simulink model "CF012A_GmStrtStop"  (R2013b)
settings: Solver=FixedStepDiscrete  SolverMode=SingleTasking  StartTime=0.0  StopTime=1  FixedStep=0.002  RelTol=1e-3
values from neighbouring files (symbols this model uses):
  CNV100MICROSECTOMILLISEC_MILLISECPERCNT_F32 = DataDict.Constant    [CF012A_GmStrtStop_DataDict.m]
  DISMOD_CNT_U08 = DataDict.Constant    [CF012A_GmStrtStop_DataDict.m]
  DISMODRATE_ULSPERSEC_F32 = DataDict.Constant    [CF012A_GmStrtStop_DataDict.m]
  FLTMOD_CNT_U08 = DataDict.Constant    [CF012A_GmStrtStop_DataDict.m]
  GmStrtStopEna = DataDict.Calibration    [CF012A_GmStrtStop_DataDict.m]
  GmStrtStopFltRateLim = DataDict.Calibration    [CF012A_GmStrtStop_DataDict.m]
  GmStrtStopMod1ToStopRateLim = DataDict.Calibration    [CF012A_GmStrtStop_DataDict.m]
  GmStrtStopNormRateLim = DataDict.Calibration    [CF012A_GmStrtStop_DataDict.m]
  GmStrtStopNormToMod1RateLim = DataDict.Calibration    [CF012A_GmStrtStop_DataDict.m]
  GmStrtStopStopAndMod2RateLim = DataDict.Calibration    [CF012A_GmStrtStop_DataDict.m]
  GmStrtStopStopMod1Tmr = DataDict.Calibration    [CF012A_GmStrtStop_DataDict.m]
  GmStrtStopStopMod2Tmr = DataDict.Calibration    [CF012A_GmStrtStop_DataDict.m]
  MOD1_CNT_U08 = DataDict.Constant    [CF012A_GmStrtStop_DataDict.m]
  MOD2_CNT_U08 = DataDict.Constant    [CF012A_GmStrtStop_DataDict.m]
  NORMMOD_CNT_U08 = DataDict.Constant    [CF012A_GmStrtStop_DataDict.m]
  STOPMOD_CNT_U08 = DataDict.Constant    [CF012A_GmStrtStop_DataDict.m]
  STRTSTOPRATEHILIM_ULSPERSEC_F32 = DataDict.Constant    [CF012A_GmStrtStop_DataDict.m]
  STRTSTOPRATELOWRLIM_ULSPERSEC_F32 = DataDict.Constant    [CF012A_GmStrtStop_DataDict.m]
  STRTSTOPSCAHILIM_ULS_F32 = DataDict.Constant    [CF012A_GmStrtStop_DataDict.m]
  STRTSTOPSCALOWRLIM_ULS_F32 = DataDict.Constant    [CF012A_GmStrtStop_DataDict.m]
undefined symbols (not defined in the file or in its folder): u2, u3, u4, u5
libraries: FixdToFloat x2, NxtrLim x2, simulink x2
(part 4 of 4)

== system CF012A_GmStrtStop/GmStrtStop/GmStrtStopPer1/Inter1ToStopModFlg/RefTi ==
  Action Port : ActionPort  ActionType=else
  Constant13 : Constant  RequirementInfo={} %GIDa_ee595446_fddf_49fb_8bdf_b7998be5b5f2  Value=false  OutDataTypeStr=boolean
      settings: AttributesFormatString=%<OutDataTypeStr>
  CopyRight2 : Subsystem  Description=|  mask(Copyright Information){none=on}
      | Copyright info block.                                               
      |                                                                     
      | Place copyright information at the top of every subsystem in design.
      mask prompts: none "No parameters"
      mask help: Place copyright information at the top of every subsystem in design.
      mask Display:
      | NxtrConf = 'Nexteer Confidential';
      | 
      | sys = bdroot; %handle for the current model ("system")
      | first = get_param(sys,'Created');
      | if(isempty(first))
      |     first = datestr(now,'yyyy');
      | else
      |     first = first(end-3:end);  %year is last four digits
      | end
      | 
      | last = get_param(sys,'LastModifiedDate');
      | if isempty(last)
      |     last = datestr(now,'yyyy');
      | else
      |     last = last(end-3:end);
      | end
      | 
      | if strcmp(first,last)
      |     fprintf('%s -- Copyright %s Nexteer',NxtrConf,first)
      | else
      |     fprintf('%s -- %s%s- %s Nexteer',NxtrConf,char(169),first,last)
      | end
  Data Store Write9 : DataStoreWrite  DataStoreName=Mod1RefTmr
  GetRefTmr100MicroSec32bit : Subsystem
  TmrElpsdThd : Outport
  wires:
  GetRefTmr100MicroSec32bit/1(RefTmr) -> Data Store Write9/1
  Constant13/1 -> TmrElpsdThd/1

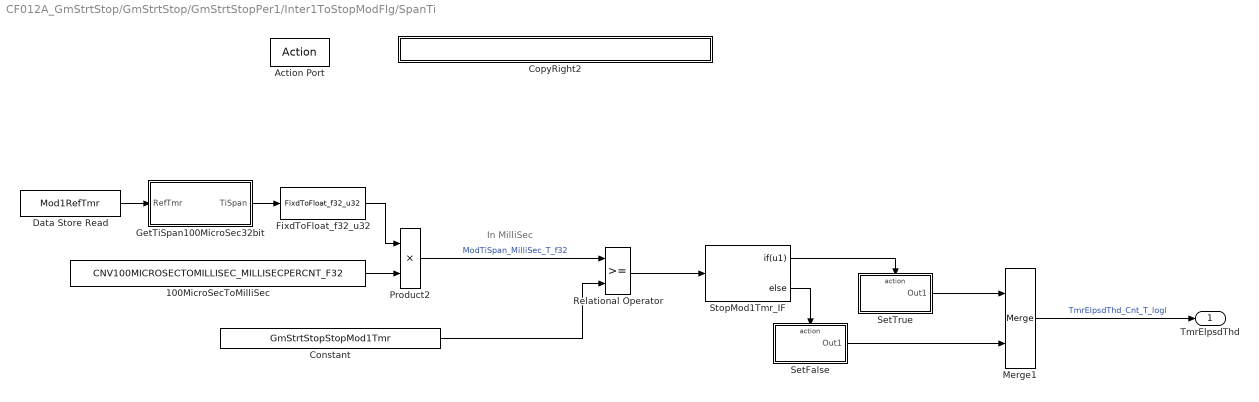
== system CF012A_GmStrtStop/GmStrtStop/GmStrtStopPer1/Inter1ToStopModFlg/SpanTi ==
  note: In MilliSec
  Action Port : ActionPort  ActionType=then
  100MicroSecToMilliSec : Constant  RequirementInfo="{'linktype_rmi_doors' '0000c6e0 (/GM T1XX/SubSystem Specifications/Customer Functions/CF012 12V Start Stop)' '#149' 'true' 'REQ:  149' '' } %GIDa_f27a5255_6b96_489d_8647_639b65e7e1e3"  Value=CNV100MICROSECTOMILLISEC_MILLISECPERCNT_F32
  Constant : Constant  RequirementInfo="{'linktype_rmi_doors' '0000c6e0 (/GM T1XX/SubSystem Specifications/Customer Functions/CF012 12V Start Stop)' '#149' 'true' 'REQ:  149' '' } %GIDa_161a89a7_a936_46ad_9e50_4b6beac1caa8"  Value=GmStrtStopStopMod1Tmr
  CopyRight2 : Subsystem  Description=|  mask(Copyright Information){none=on}
      | Copyright info block.                                               
      |                                                                     
      | Place copyright information at the top of every subsystem in design.
      mask prompts: none "No parameters"
      mask help: Place copyright information at the top of every subsystem in design.
      mask Display:
      | NxtrConf = 'Nexteer Confidential';
      | 
      | sys = bdroot; %handle for the current model ("system")
      | first = get_param(sys,'Created');
      | if(isempty(first))
      |     first = datestr(now,'yyyy');
      | else
      |     first = first(end-3:end);  %year is last four digits
      | end
      | 
      | last = get_param(sys,'LastModifiedDate');
      | if isempty(last)
      |     last = datestr(now,'yyyy');
      | else
      |     last = last(end-3:end);
      | end
      | 
      | if strcmp(first,last)
      |     fprintf('%s -- Copyright %s Nexteer',NxtrConf,first)
      | else
      |     fprintf('%s -- %s%s- %s Nexteer',NxtrConf,char(169),first,last)
      | end
  Data Store Read : DataStoreRead  RequirementInfo="{'linktype_rmi_doors' '0000c6e0 (/GM T1XX/SubSystem Specifications/Customer Functions/CF012 12V Start Stop)' '#149' 'true' 'REQ:  149' '' } %GIDa_f243752d_cd64_4ade_bc30_06d78740bec9"  DataStoreName=Mod1RefTmr
  FixdToFloat_f32_u32 : FixdToFloat/FixdToFloat_f32_u32  RequirementInfo="{'linktype_rmi_doors' '0000c6e0 (/GM T1XX/SubSystem Specifications/Customer Functions/CF012 12V Start Stop)' '#149' 'true' 'REQ:  149' '' } %GIDa_724a14fd_bedc_4ae1_8651_07fb98cb7006"  Param1=0
  GetTiSpan100MicroSec32bit : Subsystem  RequirementInfo="{'linktype_rmi_doors' '0000c6e0 (/GM T1XX/SubSystem Specifications/Customer Functions/CF012 12V Start Stop)' '#149' 'true' 'REQ:  149' '' } %GIDa_42f2edbe_6506_45bf_bc5f_21ff22e5da44"
  Merge1 : Merge  RequirementInfo="{'linktype_rmi_doors' '0000c6e0 (/GM T1XX/SubSystem Specifications/Customer Functions/CF012 12V Start Stop)' '#149' 'true' 'REQ:  149' '' } %GIDa_b6f22ad7_a1b8_4e7a_82f9_c53496e4294b"
  Product2 : Product  RequirementInfo="{'linktype_rmi_doors' '0000c6e0 (/GM T1XX/SubSystem Specifications/Customer Functions/CF012 12V Start Stop)' '#149' 'true' 'REQ:  149' '' } %GIDa_358ce13a_3b2a_451b_80f1_72e22c5f1708"
  Relational Operator : RelationalOperator  RequirementInfo="{'linktype_rmi_doors' '0000c6e0 (/GM T1XX/SubSystem Specifications/Customer Functions/CF012 12V Start Stop)' '#149' 'true' 'REQ:  149' '' } %GIDa_e7de6d6e_7f4c_4fc6_98dc_b2abb4573d8c"  OutDataTypeStr=boolean
  SetFalse : Subsystem  RequirementInfo="{'linktype_rmi_doors' '0000c6e0 (/GM T1XX/SubSystem Specifications/Customer Functions/CF012 12V Start Stop)' '#149' 'true' 'REQ:  149' '' } %GIDa_d7f0596c_8f68_4a27_b553_110820238b8a"  TreatAsAtomicUnit=on
  SetTrue : Subsystem  RequirementInfo="{'linktype_rmi_doors' '0000c6e0 (/GM T1XX/SubSystem Specifications/Customer Functions/CF012 12V Start Stop)' '#149' 'true' 'REQ:  149' '' } %GIDa_3df73667_32db_41d3_8694_836724889a59"  TreatAsAtomicUnit=on
  StopMod1Tmr_IF : If  RequirementInfo="{'linktype_rmi_doors' '0000c6e0 (/GM T1XX/SubSystem Specifications/Customer Functions/CF012 12V Start Stop)' '#149' 'true' 'REQ:  149' '' } %GIDa_ab1d4f5e_890c_4780_96ee_c57598ab3683"  IfExpression=u1
  TmrElpsdThd : Outport  RequirementInfo="{'linktype_rmi_doors' '0000c6e0 (/GM T1XX/SubSystem Specifications/Customer Functions/CF012 12V Start Stop)' '#149' 'true' 'REQ:  149' '' } %GIDa_6efc0186_5b61_45a8_8aa0_b92fa27113a3"
  wires:
  Data Store Read/1 -> GetTiSpan100MicroSec32bit/1(RefTmr)
  Merge1/1 -> TmrElpsdThd/1  "TmrElpsdThd_Cnt_T_logl"
  GetTiSpan100MicroSec32bit/1(TiSpan) -> FixdToFloat_f32_u32/1
  Relational Operator/1 -> StopMod1Tmr_IF/1
  SetTrue/1(Out1) -> Merge1/1
  SetFalse/1(Out1) -> Merge1/2
  StopMod1Tmr_IF/1 -> SetTrue/Action
  StopMod1Tmr_IF/2 -> SetFalse/Action
  100MicroSecToMilliSec/1 -> Product2/2
  FixdToFloat_f32_u32/1 -> Product2/1
  Product2/1 -> Relational Operator/1  "ModTiSpan_MilliSec_T_f32"
  Constant/1 -> Relational Operator/2

== system CF012A_GmStrtStop/GmStrtStop/GmStrtStopPer1/Inter2ToStopModFlg/CopyRight2 ==

== system CF012A_GmStrtStop/GmStrtStop/GmStrtStopPer1/Inter2ToStopModFlg/RefTi ==
  Action Port : ActionPort  ActionType=else
  Constant13 : Constant  RequirementInfo={} %GIDa_2f60d0b6_d859_47c7_824c_82648ed235eb  Value=false  OutDataTypeStr=boolean
      settings: AttributesFormatString=%<OutDataTypeStr>
  CopyRight2 : Subsystem  Description=|  mask(Copyright Information){none=on}
      | Copyright info block.                                               
      |                                                                     
      | Place copyright information at the top of every subsystem in design.
      mask prompts: none "No parameters"
      mask help: Place copyright information at the top of every subsystem in design.
      mask Display:
      | NxtrConf = 'Nexteer Confidential';
      | 
      | sys = bdroot; %handle for the current model ("system")
      | first = get_param(sys,'Created');
      | if(isempty(first))
      |     first = datestr(now,'yyyy');
      | else
      |     first = first(end-3:end);  %year is last four digits
      | end
      | 
      | last = get_param(sys,'LastModifiedDate');
      | if isempty(last)
      |     last = datestr(now,'yyyy');
      | else
      |     last = last(end-3:end);
      | end
      | 
      | if strcmp(first,last)
      |     fprintf('%s -- Copyright %s Nexteer',NxtrConf,first)
      | else
      |     fprintf('%s -- %s%s- %s Nexteer',NxtrConf,char(169),first,last)
      | end
  Data Store Write9 : DataStoreWrite  DataStoreName=Mod2RefTmr
  GetRefTmr100MicroSec32bit : Subsystem
  TmrElpsdThd : Outport
  wires:
  Constant13/1 -> TmrElpsdThd/1
  GetRefTmr100MicroSec32bit/1(RefTmr) -> Data Store Write9/1

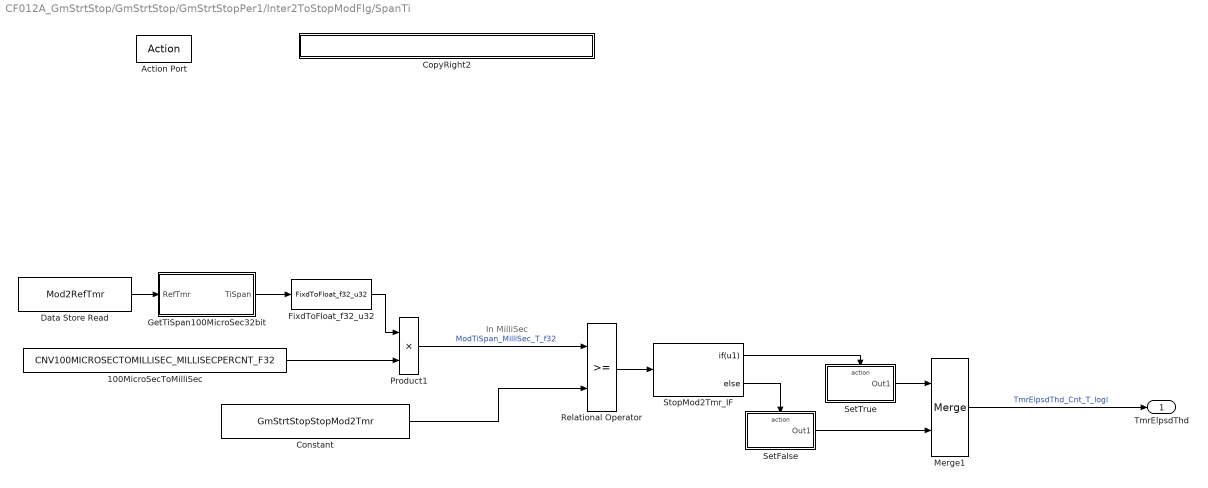
== system CF012A_GmStrtStop/GmStrtStop/GmStrtStopPer1/Inter2ToStopModFlg/SpanTi ==
  note: In MilliSec
  Action Port : ActionPort  ActionType=then
  100MicroSecToMilliSec : Constant  Value=CNV100MICROSECTOMILLISEC_MILLISECPERCNT_F32
  Constant : Constant  RequirementInfo={} %GIDa_5b9b31eb_6e21_4040_a5c7_63bbbbf883bd  Value=GmStrtStopStopMod2Tmr
  CopyRight2 : Subsystem  Description=|  mask(Copyright Information){none=on}
      | Copyright info block.                                               
      |                                                                     
      | Place copyright information at the top of every subsystem in design.
      mask prompts: none "No parameters"
      mask help: Place copyright information at the top of every subsystem in design.
      mask Display:
      | NxtrConf = 'Nexteer Confidential';
      | 
      | sys = bdroot; %handle for the current model ("system")
      | first = get_param(sys,'Created');
      | if(isempty(first))
      |     first = datestr(now,'yyyy');
      | else
      |     first = first(end-3:end);  %year is last four digits
      | end
      | 
      | last = get_param(sys,'LastModifiedDate');
      | if isempty(last)
      |     last = datestr(now,'yyyy');
      | else
      |     last = last(end-3:end);
      | end
      | 
      | if strcmp(first,last)
      |     fprintf('%s -- Copyright %s Nexteer',NxtrConf,first)
      | else
      |     fprintf('%s -- %s%s- %s Nexteer',NxtrConf,char(169),first,last)
      | end
  Data Store Read : DataStoreRead  DataStoreName=Mod2RefTmr
  FixdToFloat_f32_u32 : FixdToFloat/FixdToFloat_f32_u32  Param1=0
  GetTiSpan100MicroSec32bit : Subsystem
  Merge1 : Merge
  Product1 : Product
  Relational Operator : RelationalOperator  OutDataTypeStr=boolean
  SetFalse : Subsystem  TreatAsAtomicUnit=on
  SetTrue : Subsystem  TreatAsAtomicUnit=on
  StopMod2Tmr_IF : If  IfExpression=u1
  TmrElpsdThd : Outport
  wires:
  StopMod2Tmr_IF/2 -> SetFalse/Action
  SetFalse/1(Out1) -> Merge1/2
  SetTrue/1(Out1) -> Merge1/1
  StopMod2Tmr_IF/1 -> SetTrue/Action
  Relational Operator/1 -> StopMod2Tmr_IF/1
  GetTiSpan100MicroSec32bit/1(TiSpan) -> FixdToFloat_f32_u32/1
  Merge1/1 -> TmrElpsdThd/1  "TmrElpsdThd_Cnt_T_logl"
  Data Store Read/1 -> GetTiSpan100MicroSec32bit/1(RefTmr)
  FixdToFloat_f32_u32/1 -> Product1/1
  100MicroSecToMilliSec/1 -> Product1/2
  Product1/1 -> Relational Operator/1  "ModTiSpan_MilliSec_T_f32"
  Constant/1 -> Relational Operator/2

== system CF012A_GmStrtStop/GmStrtStop/GmStrtStopPer1/PassDtrmnRateRes/CopyRight2 ==

== system CF012A_GmStrtStop/GmStrtStop/GmStrtStopPer1/DtrmnPrevActSt/PassLastSt/CopyRight2 ==

== system CF012A_GmStrtStop/GmStrtStop/GmStrtStopPer1/DtrmnPrevActSt/PassPrevLoopRes/CopyRight2 ==

== system CF012A_GmStrtStop/GmStrtStop/GmStrtStopPer1/DtrmnRateLim/DoNothing/CopyRight2 ==

== system CF012A_GmStrtStop/GmStrtStop/GmStrtStopPer1/DtrmnRateLim/FltMod/CopyRight2 ==

== system CF012A_GmStrtStop/GmStrtStop/GmStrtStopPer1/DtrmnRateLim/Inter1Mod/CopyRight2 ==

== system CF012A_GmStrtStop/GmStrtStop/GmStrtStopPer1/DtrmnRateLim/Inter1Mod/THEN1 ==
  note: Change Log:
      | Oct 12, 2012  Created by Kevin Derry as a 1-input, 1-output block
      | Nov 30, 2012  dynamically configurable for 1 to 5 ports.
  note: Do not modify these blocks manually.  They
      | are generated programatically.  Changing the
      | number of blocks available or their names requires
      | corresponding changes to Callback and Initialization
      | routines.
      |
      | Do not change the "Display" tab of mask editor.  The
      | outport names are created programatically in the
      | "Initialize" section.
  In1 : Inport
  Action Port : ActionPort  ActionType=then
  In{2..5} (4 alike) : Ground
  Out{2..5} (4 alike) : Terminator
  Out1 : Outport
  wires:
  In1/1 -> Out1/1
  In2/1 -> Out2/1
  In3/1 -> Out3/1
  In4/1 -> Out4/1
  In5/1 -> Out5/1

== system CF012A_GmStrtStop/GmStrtStop/GmStrtStopPer1/DtrmnRateLim/Inter1Mod/THEN2 ==
  note: Do not modify these blocks manually.  They
      | are generated programatically.  Changing the
      | number of blocks available or their names requires
      | corresponding changes to Callback and Initialization
      | routines.
      |
      | Do not change the "Display" tab of mask editor.  The
      | outport names are created programatically in the
      | "Initialize" section.
  note: Change Log:
      | Oct 12, 2012  Created by Kevin Derry as a 1-input, 1-output block
      | Nov 30, 2012  dynamically configurable for 1 to 5 ports.
  In1 : Inport
  Action Port : ActionPort  ActionType=elseif
  In{2..5} (4 alike) : Ground
  Out{2..5} (4 alike) : Terminator
  Out1 : Outport
  wires:
  In5/1 -> Out5/1
  In4/1 -> Out4/1
  In3/1 -> Out3/1
  In2/1 -> Out2/1
  In1/1 -> Out1/1

== system CF012A_GmStrtStop/GmStrtStop/GmStrtStopPer1/DtrmnRateLim/Inter1Mod/THEN3 ==
  note: Change Log:
      | Oct 12, 2012  Created by Kevin Derry as a 1-input, 1-output block
      | Nov 30, 2012  dynamically configurable for 1 to 5 ports.
  note: Do not modify these blocks manually.  They
      | are generated programatically.  Changing the
      | number of blocks available or their names requires
      | corresponding changes to Callback and Initialization
      | routines.
      |
      | Do not change the "Display" tab of mask editor.  The
      | outport names are created programatically in the
      | "Initialize" section.
  In1 : Inport
  Action Port : ActionPort  ActionType=else
  In{2..5} (4 alike) : Ground
  Out{2..5} (4 alike) : Terminator
  Out1 : Outport
  wires:
  In1/1 -> Out1/1
  In2/1 -> Out2/1
  In3/1 -> Out3/1
  In4/1 -> Out4/1
  In5/1 -> Out5/1

== system CF012A_GmStrtStop/GmStrtStop/GmStrtStopPer1/DtrmnRateLim/Inter2Mod/CopyRight2 ==

== system CF012A_GmStrtStop/GmStrtStop/GmStrtStopPer1/DtrmnRateLim/Inter2Mod/THEN1 ==
  note: Change Log:
      | Oct 12, 2012  Created by Kevin Derry as a 1-input, 1-output block
      | Nov 30, 2012  dynamically configurable for 1 to 5 ports.
  note: Do not modify these blocks manually.  They
      | are generated programatically.  Changing the
      | number of blocks available or their names requires
      | corresponding changes to Callback and Initialization
      | routines.
      |
      | Do not change the "Display" tab of mask editor.  The
      | outport names are created programatically in the
      | "Initialize" section.
  In1 : Inport
  Action Port : ActionPort  ActionType=then
  In{2..5} (4 alike) : Ground
  Out{2..5} (4 alike) : Terminator
  Out1 : Outport
  wires:
  In1/1 -> Out1/1
  In2/1 -> Out2/1
  In3/1 -> Out3/1
  In4/1 -> Out4/1
  In5/1 -> Out5/1

== system CF012A_GmStrtStop/GmStrtStop/GmStrtStopPer1/DtrmnRateLim/Inter2Mod/THEN2 ==
  note: Do not modify these blocks manually.  They
      | are generated programatically.  Changing the
      | number of blocks available or their names requires
      | corresponding changes to Callback and Initialization
      | routines.
      |
      | Do not change the "Display" tab of mask editor.  The
      | outport names are created programatically in the
      | "Initialize" section.
  note: Change Log:
      | Oct 12, 2012  Created by Kevin Derry as a 1-input, 1-output block
      | Nov 30, 2012  dynamically configurable for 1 to 5 ports.
  In1 : Inport
  Action Port : ActionPort  ActionType=elseif
  In{2..5} (4 alike) : Ground
  Out{2..5} (4 alike) : Terminator
  Out1 : Outport
  wires:
  In5/1 -> Out5/1
  In4/1 -> Out4/1
  In3/1 -> Out3/1
  In2/1 -> Out2/1
  In1/1 -> Out1/1

== system CF012A_GmStrtStop/GmStrtStop/GmStrtStopPer1/DtrmnRateLim/Inter2Mod/THEN3 ==
  note: Change Log:
      | Oct 12, 2012  Created by Kevin Derry as a 1-input, 1-output block
      | Nov 30, 2012  dynamically configurable for 1 to 5 ports.
  note: Do not modify these blocks manually.  They
      | are generated programatically.  Changing the
      | number of blocks available or their names requires
      | corresponding changes to Callback and Initialization
      | routines.
      |
      | Do not change the "Display" tab of mask editor.  The
      | outport names are created programatically in the
      | "Initialize" section.
  In1 : Inport
  Action Port : ActionPort  ActionType=else
  In{2..5} (4 alike) : Ground
  Out{2..5} (4 alike) : Terminator
  Out1 : Outport
  wires:
  In1/1 -> Out1/1
  In2/1 -> Out2/1
  In3/1 -> Out3/1
  In4/1 -> Out4/1
  In5/1 -> Out5/1

== system CF012A_GmStrtStop/GmStrtStop/GmStrtStopPer1/DtrmnRateLim/NormMod/CopyRight2 ==

== system CF012A_GmStrtStop/GmStrtStop/GmStrtStopPer1/DtrmnRateLim/NormMod/THEN3 ==
  note: Change Log:
      | Oct 12, 2012  Created by Kevin Derry as a 1-input, 1-output block
      | Nov 30, 2012  dynamically configurable for 1 to 5 ports.
  note: Do not modify these blocks manually.  They
      | are generated programatically.  Changing the
      | number of blocks available or their names requires
      | corresponding changes to Callback and Initialization
      | routines.
      |
      | Do not change the "Display" tab of mask editor.  The
      | outport names are created programatically in the
      | "Initialize" section.
  In1 : Inport
  Action Port : ActionPort  ActionType=then
  In{2..5} (4 alike) : Ground
  Out{2..5} (4 alike) : Terminator
  Out1 : Outport
  wires:
  In1/1 -> Out1/1
  In2/1 -> Out2/1
  In3/1 -> Out3/1
  In4/1 -> Out4/1
  In5/1 -> Out5/1

== system CF012A_GmStrtStop/GmStrtStop/GmStrtStopPer1/DtrmnRateLim/NormMod/THEN4 ==
  note: Do not modify these blocks manually.  They
      | are generated programatically.  Changing the
      | number of blocks available or their names requires
      | corresponding changes to Callback and Initialization
      | routines.
      |
      | Do not change the "Display" tab of mask editor.  The
      | outport names are created programatically in the
      | "Initialize" section.
  note: Change Log:
      | Oct 12, 2012  Created by Kevin Derry as a 1-input, 1-output block
      | Nov 30, 2012  dynamically configurable for 1 to 5 ports.
  In1 : Inport
  Action Port : ActionPort  ActionType=else
  In{2..5} (4 alike) : Ground
  Out{2..5} (4 alike) : Terminator
  Out1 : Outport
  wires:
  In5/1 -> Out5/1
  In4/1 -> Out4/1
  In3/1 -> Out3/1
  In2/1 -> Out2/1
  In1/1 -> Out1/1

== system CF012A_GmStrtStop/GmStrtStop/GmStrtStopPer1/DtrmnRateLim/StopMod/CopyRight2 ==

== system CF012A_GmStrtStop/GmStrtStop/GmStrtStopPer1/DtrmnRateLim/StopMod/THEN1 ==
  note: Change Log:
      | Oct 12, 2012  Created by Kevin Derry as a 1-input, 1-output block
      | Nov 30, 2012  dynamically configurable for 1 to 5 ports.
  note: Do not modify these blocks manually.  They
      | are generated programatically.  Changing the
      | number of blocks available or their names requires
      | corresponding changes to Callback and Initialization
      | routines.
      |
      | Do not change the "Display" tab of mask editor.  The
      | outport names are created programatically in the
      | "Initialize" section.
  In1 : Inport
  Action Port : ActionPort  ActionType=then
  In{2..5} (4 alike) : Ground
  Out{2..5} (4 alike) : Terminator
  Out1 : Outport
  wires:
  In1/1 -> Out1/1
  In2/1 -> Out2/1
  In3/1 -> Out3/1
  In4/1 -> Out4/1
  In5/1 -> Out5/1

== system CF012A_GmStrtStop/GmStrtStop/GmStrtStopPer1/DtrmnRateLim/StopMod/THEN4 ==
  note: Do not modify these blocks manually.  They
      | are generated programatically.  Changing the
      | number of blocks available or their names requires
      | corresponding changes to Callback and Initialization
      | routines.
      |
      | Do not change the "Display" tab of mask editor.  The
      | outport names are created programatically in the
      | "Initialize" section.
  note: Change Log:
      | Oct 12, 2012  Created by Kevin Derry as a 1-input, 1-output block
      | Nov 30, 2012  dynamically configurable for 1 to 5 ports.
  In1 : Inport
  Action Port : ActionPort  ActionType=elseif
  In{2..5} (4 alike) : Ground
  Out{2..5} (4 alike) : Terminator
  Out1 : Outport
  wires:
  In5/1 -> Out5/1
  In4/1 -> Out4/1
  In3/1 -> Out3/1
  In2/1 -> Out2/1
  In1/1 -> Out1/1

== system CF012A_GmStrtStop/GmStrtStop/GmStrtStopPer1/DtrmnRateLim/StopMod/THEN5 ==
  note: Change Log:
      | Oct 12, 2012  Created by Kevin Derry as a 1-input, 1-output block
      | Nov 30, 2012  dynamically configurable for 1 to 5 ports.
  note: Do not modify these blocks manually.  They
      | are generated programatically.  Changing the
      | number of blocks available or their names requires
      | corresponding changes to Callback and Initialization
      | routines.
      |
      | Do not change the "Display" tab of mask editor.  The
      | outport names are created programatically in the
      | "Initialize" section.
  In1 : Inport
  Action Port : ActionPort  ActionType=else
  In{2..5} (4 alike) : Ground
  Out{2..5} (4 alike) : Terminator
  Out1 : Outport
  wires:
  In1/1 -> Out1/1
  In2/1 -> Out2/1
  In3/1 -> Out3/1
  In4/1 -> Out4/1
  In5/1 -> Out5/1

== system CF012A_GmStrtStop/GmStrtStop/GmStrtStopPer1/Inter1ToStopModFlg/RefTi/CopyRight2 ==

== system CF012A_GmStrtStop/GmStrtStop/GmStrtStopPer1/Inter1ToStopModFlg/RefTi/GetRefTmr100MicroSec32bit ==
  note: Created Aug 18, 2015
      | Modified Oct 21, 2015
      | Modified Oct 30, 2015
      | Kevin Derry
  note: GetRefTmr100MicroSec32bit
  note: Wrap-to-zero
  note: counts
  note: microseconds
  note: seconds
  note: 1 count = 100 uSec
  CopyRight2 : Subsystem  Description=|  mask(Copyright Information){none=on}
      | Copyright info block.                                               
      |                                                                     
      | Place copyright information at the top of every subsystem in design.
      mask prompts: none "No parameters"
      mask help: Place copyright information at the top of every subsystem in design.
      mask Display:
      | NxtrConf = 'Nexteer Confidential';
      | 
      | sys = bdroot; %handle for the current model ("system")
      | first = get_param(sys,'Created');
      | if(isempty(first))
      |     first = datestr(now,'yyyy');
      | else
      |     first = first(end-3:end);  %year is last four digits
      | end
      | 
      | last = get_param(sys,'LastModifiedDate');
      | if isempty(last)
      |     last = datestr(now,'yyyy');
      | else
      |     last = last(end-3:end);
      | end
      | 
      | if strcmp(first,last)
      |     fprintf('%s -- Copyright %s Nexteer',NxtrConf,first)
      | else
      |     fprintf('%s -- %s%s- %s Nexteer',NxtrConf,char(169),first,last)
      | end
  Count per uSec : Constant  Value=0.01
  Data Store Read1 : DataStoreRead  DataStoreName=SimnTi
  Data Type Conversion1 : DataTypeConversion  OutDataTypeStr=uint32
  Divide1 : Product  Inputs=**
  Divide2 : Product  Inputs=*/
  Max Counts : Constant  Value=2^32-1
  Product1 : Product
  Product2 : Product
  Rounding : Rounding
  Subtract1 : Sum  Inputs=+-
  uSec per Sec : Constant  Value=1000000
  RefTmr : Outport
  wires:
  Data Store Read1/1 -> Product1/1
  Data Type Conversion1/1 -> RefTmr/1
  uSec per Sec/1 -> Product1/2
  Count per uSec/1 -> Divide1/2
  Product1/1 -> Divide1/1
  Divide1/1 -> Subtract1/1, Divide2/1
  Max Counts/1 -> Product2/2, Divide2/2
  Divide2/1 -> Rounding/1
  Rounding/1 -> Product2/1
  Subtract1/1 -> Data Type Conversion1/1
  Product2/1 -> Subtract1/2

== system CF012A_GmStrtStop/GmStrtStop/GmStrtStopPer1/Inter1ToStopModFlg/SpanTi/CopyRight2 ==

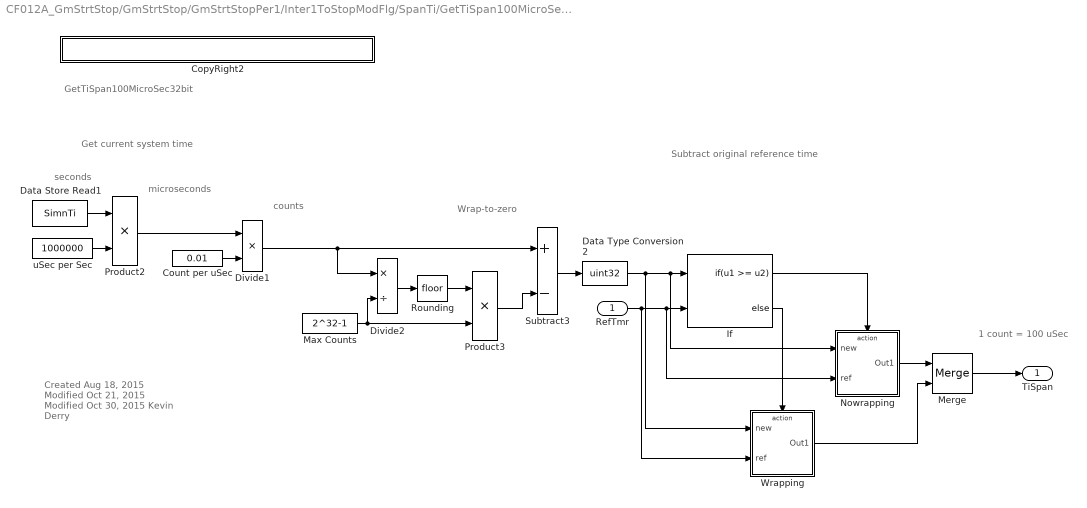
== system CF012A_GmStrtStop/GmStrtStop/GmStrtStopPer1/Inter1ToStopModFlg/SpanTi/GetTiSpan100MicroSec32bit ==
  note: Created Aug 18, 2015
      | Modified Oct 21, 2015
      | Modified Oct 30, 2015
      | Kevin Derry
  note: GetTiSpan100MicroSec32bit
  note: Get current system time
  note: 1 count = 100 uSec
  note: Wrap-to-zero
  note: counts
  note: microseconds
  note: seconds
  note: Subtract original reference time
  RefTmr : Inport
  CopyRight2 : Subsystem  Description=|  mask(Copyright Information){none=on}
      | Copyright info block.                                               
      |                                                                     
      | Place copyright information at the top of every subsystem in design.
      mask prompts: none "No parameters"
      mask help: Place copyright information at the top of every subsystem in design.
      mask Display:
      | NxtrConf = 'Nexteer Confidential';
      | 
      | sys = bdroot; %handle for the current model ("system")
      | first = get_param(sys,'Created');
      | if(isempty(first))
      |     first = datestr(now,'yyyy');
      | else
      |     first = first(end-3:end);  %year is last four digits
      | end
      | 
      | last = get_param(sys,'LastModifiedDate');
      | if isempty(last)
      |     last = datestr(now,'yyyy');
      | else
      |     last = last(end-3:end);
      | end
      | 
      | if strcmp(first,last)
      |     fprintf('%s -- Copyright %s Nexteer',NxtrConf,first)
      | else
      |     fprintf('%s -- %s%s- %s Nexteer',NxtrConf,char(169),first,last)
      | end
  Count per uSec : Constant  Value=0.01
  Data Store Read1 : DataStoreRead  DataStoreName=SimnTi
  Data Type Conversion2 : DataTypeConversion  OutDataTypeStr=uint32
  Divide1 : Product  Inputs=**
  Divide2 : Product  Inputs=*/
  If : If  NumInputs=2  IfExpression=u1 >= u2
  Max Counts : Constant  Value=2^32-1
  Merge : Merge
  Nowrapping : Subsystem  TreatAsAtomicUnit=on
  Product2 : Product
  Product3 : Product
  Rounding : Rounding
  Subtract3 : Sum  Inputs=+-
  Wrapping : Subsystem  TreatAsAtomicUnit=on
  uSec per Sec : Constant  Value=1000000
  TiSpan : Outport
  wires:
  Data Type Conversion2/1 -> Wrapping/1(new), Nowrapping/1(new), If/1
  RefTmr/1 -> Wrapping/2(ref), Nowrapping/2(ref), If/2
  Merge/1 -> TiSpan/1
  uSec per Sec/1 -> Product2/2
  Count per uSec/1 -> Divide1/2
  Data Store Read1/1 -> Product2/1
  Product2/1 -> Divide1/1
  Divide1/1 -> Subtract3/1, Divide2/1
  Max Counts/1 -> Product3/2, Divide2/2
  Divide2/1 -> Rounding/1
  Rounding/1 -> Product3/1
  Subtract3/1 -> Data Type Conversion2/1
  Product3/1 -> Subtract3/2
  If/1 -> Nowrapping/Action
  If/2 -> Wrapping/Action
  Nowrapping/1(Out1) -> Merge/1
  Wrapping/1(Out1) -> Merge/2

== system CF012A_GmStrtStop/GmStrtStop/GmStrtStopPer1/Inter1ToStopModFlg/SpanTi/SetFalse ==
  Action Port : ActionPort  ActionType=else
  Constant1 : Constant  RequirementInfo={} %GIDa_daf20740_f42b_4a36_be92_178642fae00b  Value=false  OutDataTypeStr=boolean
      settings: AttributesFormatString=%<OutDataTypeStr>
  CopyRight2 : Subsystem  Description=|  mask(Copyright Information){none=on}
      | Copyright info block.                                               
      |                                                                     
      | Place copyright information at the top of every subsystem in design.
      mask prompts: none "No parameters"
      mask help: Place copyright information at the top of every subsystem in design.
      mask Display:
      | NxtrConf = 'Nexteer Confidential';
      | 
      | sys = bdroot; %handle for the current model ("system")
      | first = get_param(sys,'Created');
      | first = first(end-3:end);  %year is last four digits
      | 
      | last = get_param(sys,'LastModifiedDate');
      | if isempty(last)
      |     last = datestr(now,'yyyy');
      | else
      |     last = last(end-3:end);
      | end
      | 
      | if strcmp(first,last)
      |     fprintf('%s -- Copyright %s Nexteer',NxtrConf,first)
      | else
      |     fprintf('%s -- %s%s- %s Nexteer',NxtrConf,char(169),first,last)
      | end
  Out1 : Outport
  wires:
  Constant1/1 -> Out1/1

== system CF012A_GmStrtStop/GmStrtStop/GmStrtStopPer1/Inter1ToStopModFlg/SpanTi/SetTrue ==
  Action Port : ActionPort  ActionType=then
  Constant13 : Constant  RequirementInfo={} %GIDa_a9eb31fa_9104_4d56_b220_20a7652585d7  Value=true  OutDataTypeStr=boolean
      settings: AttributesFormatString=%<OutDataTypeStr>
  CopyRight2 : Subsystem  Description=|  mask(Copyright Information){none=on}
      | Copyright info block.                                               
      |                                                                     
      | Place copyright information at the top of every subsystem in design.
      mask prompts: none "No parameters"
      mask help: Place copyright information at the top of every subsystem in design.
      mask Display:
      | NxtrConf = 'Nexteer Confidential';
      | 
      | sys = bdroot; %handle for the current model ("system")
      | first = get_param(sys,'Created');
      | first = first(end-3:end);  %year is last four digits
      | 
      | last = get_param(sys,'LastModifiedDate');
      | if isempty(last)
      |     last = datestr(now,'yyyy');
      | else
      |     last = last(end-3:end);
      | end
      | 
      | if strcmp(first,last)
      |     fprintf('%s -- Copyright %s Nexteer',NxtrConf,first)
      | else
      |     fprintf('%s -- %s%s- %s Nexteer',NxtrConf,char(169),first,last)
      | end
  Out1 : Outport
  wires:
  Constant13/1 -> Out1/1

== system CF012A_GmStrtStop/GmStrtStop/GmStrtStopPer1/Inter2ToStopModFlg/RefTi/CopyRight2 ==

== system CF012A_GmStrtStop/GmStrtStop/GmStrtStopPer1/Inter2ToStopModFlg/RefTi/GetRefTmr100MicroSec32bit ==
  note: 1 count = 100 uSec
  note: seconds
  note: microseconds
  note: counts
  note: Wrap-to-zero
  note: GetRefTmr100MicroSec32bit
  note: Created Aug 18, 2015
      | Modified Oct 21, 2015
      | Modified Oct 30, 2015
      | Kevin Derry
  CopyRight2 : Subsystem  Description=|  mask(Copyright Information){none=on}
      | Copyright info block.                                               
      |                                                                     
      | Place copyright information at the top of every subsystem in design.
      mask prompts: none "No parameters"
      mask help: Place copyright information at the top of every subsystem in design.
      mask Display:
      | NxtrConf = 'Nexteer Confidential';
      | 
      | sys = bdroot; %handle for the current model ("system")
      | first = get_param(sys,'Created');
      | if(isempty(first))
      |     first = datestr(now,'yyyy');
      | else
      |     first = first(end-3:end);  %year is last four digits
      | end
      | 
      | last = get_param(sys,'LastModifiedDate');
      | if isempty(last)
      |     last = datestr(now,'yyyy');
      | else
      |     last = last(end-3:end);
      | end
      | 
      | if strcmp(first,last)
      |     fprintf('%s -- Copyright %s Nexteer',NxtrConf,first)
      | else
      |     fprintf('%s -- %s%s- %s Nexteer',NxtrConf,char(169),first,last)
      | end
  Count per uSec : Constant  Value=0.01
  Data Store Read1 : DataStoreRead  DataStoreName=SimnTi
  Data Type Conversion1 : DataTypeConversion  OutDataTypeStr=uint32
  Divide1 : Product  Inputs=**
  Divide2 : Product  Inputs=*/
  Max Counts : Constant  Value=2^32-1
  Product1 : Product
  Product2 : Product
  Rounding : Rounding
  Subtract1 : Sum  Inputs=+-
  uSec per Sec : Constant  Value=1000000
  RefTmr : Outport
  wires:
  Product2/1 -> Subtract1/2
  Subtract1/1 -> Data Type Conversion1/1
  Rounding/1 -> Product2/1
  Divide2/1 -> Rounding/1
  Max Counts/1 -> Divide2/2, Product2/2
  Divide1/1 -> Divide2/1, Subtract1/1
  Product1/1 -> Divide1/1
  Count per uSec/1 -> Divide1/2
  uSec per Sec/1 -> Product1/2
  Data Type Conversion1/1 -> RefTmr/1
  Data Store Read1/1 -> Product1/1

== system CF012A_GmStrtStop/GmStrtStop/GmStrtStopPer1/Inter2ToStopModFlg/SpanTi/CopyRight2 ==

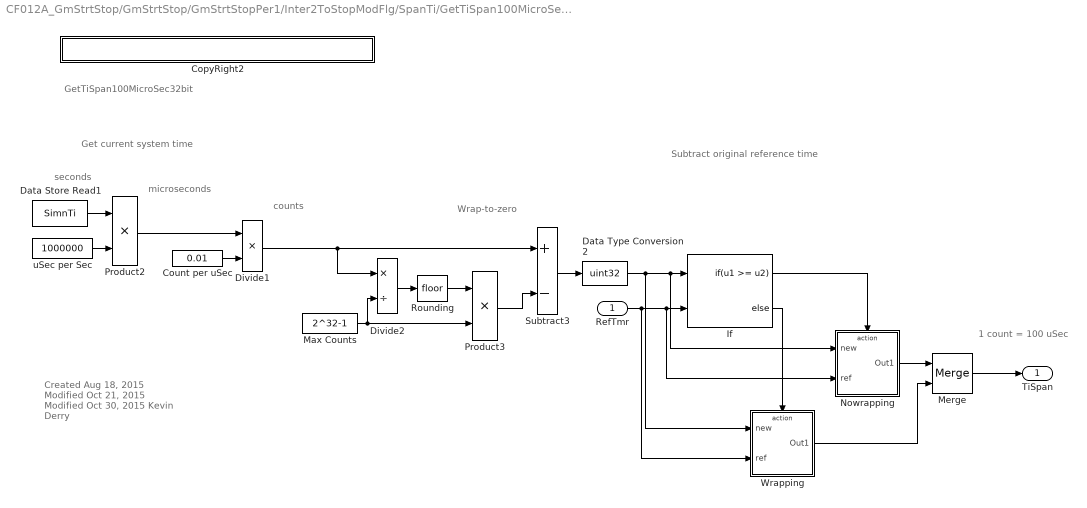
== system CF012A_GmStrtStop/GmStrtStop/GmStrtStopPer1/Inter2ToStopModFlg/SpanTi/GetTiSpan100MicroSec32bit ==
  note: Subtract original reference time
  note: seconds
  note: microseconds
  note: counts
  note: Wrap-to-zero
  note: 1 count = 100 uSec
  note: Get current system time
  note: GetTiSpan100MicroSec32bit
  note: Created Aug 18, 2015
      | Modified Oct 21, 2015
      | Modified Oct 30, 2015
      | Kevin Derry
  RefTmr : Inport
  CopyRight2 : Subsystem  Description=|  mask(Copyright Information){none=on}
      | Copyright info block.                                               
      |                                                                     
      | Place copyright information at the top of every subsystem in design.
      mask prompts: none "No parameters"
      mask help: Place copyright information at the top of every subsystem in design.
      mask Display:
      | NxtrConf = 'Nexteer Confidential';
      | 
      | sys = bdroot; %handle for the current model ("system")
      | first = get_param(sys,'Created');
      | if(isempty(first))
      |     first = datestr(now,'yyyy');
      | else
      |     first = first(end-3:end);  %year is last four digits
      | end
      | 
      | last = get_param(sys,'LastModifiedDate');
      | if isempty(last)
      |     last = datestr(now,'yyyy');
      | else
      |     last = last(end-3:end);
      | end
      | 
      | if strcmp(first,last)
      |     fprintf('%s -- Copyright %s Nexteer',NxtrConf,first)
      | else
      |     fprintf('%s -- %s%s- %s Nexteer',NxtrConf,char(169),first,last)
      | end
  Count per uSec : Constant  Value=0.01
  Data Store Read1 : DataStoreRead  DataStoreName=SimnTi
  Data Type Conversion2 : DataTypeConversion  OutDataTypeStr=uint32
  Divide1 : Product  Inputs=**
  Divide2 : Product  Inputs=*/
  If : If  NumInputs=2  IfExpression=u1 >= u2
  Max Counts : Constant  Value=2^32-1
  Merge : Merge
  Nowrapping : Subsystem  TreatAsAtomicUnit=on
  Product2 : Product
  Product3 : Product
  Rounding : Rounding
  Subtract3 : Sum  Inputs=+-
  Wrapping : Subsystem  TreatAsAtomicUnit=on
  uSec per Sec : Constant  Value=1000000
  TiSpan : Outport
  wires:
  Wrapping/1(Out1) -> Merge/2
  Nowrapping/1(Out1) -> Merge/1
  If/2 -> Wrapping/Action
  If/1 -> Nowrapping/Action
  Product3/1 -> Subtract3/2
  Subtract3/1 -> Data Type Conversion2/1
  Rounding/1 -> Product3/1
  Divide2/1 -> Rounding/1
  Max Counts/1 -> Divide2/2, Product3/2
  Divide1/1 -> Divide2/1, Subtract3/1
  Product2/1 -> Divide1/1
  Data Store Read1/1 -> Product2/1
  Count per uSec/1 -> Divide1/2
  uSec per Sec/1 -> Product2/2
  Merge/1 -> TiSpan/1
  RefTmr/1 -> If/2, Nowrapping/2(ref), Wrapping/2(ref)
  Data Type Conversion2/1 -> If/1, Nowrapping/1(new), Wrapping/1(new)

== system CF012A_GmStrtStop/GmStrtStop/GmStrtStopPer1/Inter2ToStopModFlg/SpanTi/SetFalse ==
  Action Port : ActionPort  ActionType=else
  Constant1 : Constant  RequirementInfo={} %GIDa_5a7410ee_7b51_4bf5_a69d_b85cae745ff5  Value=false  OutDataTypeStr=boolean
      settings: AttributesFormatString=%<OutDataTypeStr>
  CopyRight2 : Subsystem  Description=|  mask(Copyright Information){none=on}
      | Copyright info block.                                               
      |                                                                     
      | Place copyright information at the top of every subsystem in design.
      mask prompts: none "No parameters"
      mask help: Place copyright information at the top of every subsystem in design.
      mask Display:
      | NxtrConf = 'Nexteer Confidential';
      | 
      | sys = bdroot; %handle for the current model ("system")
      | first = get_param(sys,'Created');
      | first = first(end-3:end);  %year is last four digits
      | 
      | last = get_param(sys,'LastModifiedDate');
      | if isempty(last)
      |     last = datestr(now,'yyyy');
      | else
      |     last = last(end-3:end);
      | end
      | 
      | if strcmp(first,last)
      |     fprintf('%s -- Copyright %s Nexteer',NxtrConf,first)
      | else
      |     fprintf('%s -- %s%s- %s Nexteer',NxtrConf,char(169),first,last)
      | end
  Out1 : Outport
  wires:
  Constant1/1 -> Out1/1

== system CF012A_GmStrtStop/GmStrtStop/GmStrtStopPer1/Inter2ToStopModFlg/SpanTi/SetTrue ==
  Action Port : ActionPort  ActionType=then
  Constant13 : Constant  RequirementInfo={} %GIDa_bcd1a952_24b3_4dc8_9030_43ffd02e7b00  Value=true  OutDataTypeStr=boolean
      settings: AttributesFormatString=%<OutDataTypeStr>
  CopyRight2 : Subsystem  Description=|  mask(Copyright Information){none=on}
      | Copyright info block.                                               
      |                                                                     
      | Place copyright information at the top of every subsystem in design.
      mask prompts: none "No parameters"
      mask help: Place copyright information at the top of every subsystem in design.
      mask Display:
      | NxtrConf = 'Nexteer Confidential';
      | 
      | sys = bdroot; %handle for the current model ("system")
      | first = get_param(sys,'Created');
      | first = first(end-3:end);  %year is last four digits
      | 
      | last = get_param(sys,'LastModifiedDate');
      | if isempty(last)
      |     last = datestr(now,'yyyy');
      | else
      |     last = last(end-3:end);
      | end
      | 
      | if strcmp(first,last)
      |     fprintf('%s -- Copyright %s Nexteer',NxtrConf,first)
      | else
      |     fprintf('%s -- %s%s- %s Nexteer',NxtrConf,char(169),first,last)
      | end
  Out1 : Outport
  wires:
  Constant13/1 -> Out1/1

== system CF012A_GmStrtStop/GmStrtStop/GmStrtStopPer1/Inter1ToStopModFlg/RefTi/GetRefTmr100MicroSec32bit/CopyRight2 ==

== system CF012A_GmStrtStop/GmStrtStop/GmStrtStopPer1/Inter1ToStopModFlg/SpanTi/GetTiSpan100MicroSec32bit/CopyRight2 ==

== system CF012A_GmStrtStop/GmStrtStop/GmStrtStopPer1/Inter1ToStopModFlg/SpanTi/GetTiSpan100MicroSec32bit/Nowrapping ==
  new : Inport
  ref : Inport  Port=2
  Action Port : ActionPort  ActionType=then
  CopyRight2 : Subsystem  Description=|  mask(Copyright Information){none=on}
      | Copyright info block.                                               
      |                                                                     
      | Place copyright information at the top of every subsystem in design.
      mask prompts: none "No parameters"
      mask help: Place copyright information at the top of every subsystem in design.
      mask Display:
      | NxtrConf = 'Nexteer Confidential';
      | 
      | sys = bdroot; %handle for the current model ("system")
      | first = get_param(sys,'Created');
      | if(isempty(first))
      |     first = datestr(now,'yyyy');
      | else
      |     first = first(end-3:end);  %year is last four digits
      | end
      | 
      | last = get_param(sys,'LastModifiedDate');
      | if isempty(last)
      |     last = datestr(now,'yyyy');
      | else
      |     last = last(end-3:end);
      | end
      | 
      | if strcmp(first,last)
      |     fprintf('%s -- Copyright %s Nexteer',NxtrConf,first)
      | else
      |     fprintf('%s -- %s%s- %s Nexteer',NxtrConf,char(169),first,last)
      | end
  Subtract1 : Sum  Inputs=+-
  Out1 : Outport
  wires:
  Subtract1/1 -> Out1/1
  new/1 -> Subtract1/1
  ref/1 -> Subtract1/2

== system CF012A_GmStrtStop/GmStrtStop/GmStrtStopPer1/Inter1ToStopModFlg/SpanTi/GetTiSpan100MicroSec32bit/Wrapping ==
  new : Inport
  ref : Inport  Port=2
  Action Port : ActionPort  ActionType=else
  CopyRight2 : Subsystem  Description=|  mask(Copyright Information){none=on}
      | Copyright info block.                                               
      |                                                                     
      | Place copyright information at the top of every subsystem in design.
      mask prompts: none "No parameters"
      mask help: Place copyright information at the top of every subsystem in design.
      mask Display:
      | NxtrConf = 'Nexteer Confidential';
      | 
      | sys = bdroot; %handle for the current model ("system")
      | first = get_param(sys,'Created');
      | if(isempty(first))
      |     first = datestr(now,'yyyy');
      | else
      |     first = first(end-3:end);  %year is last four digits
      | end
      | 
      | last = get_param(sys,'LastModifiedDate');
      | if isempty(last)
      |     last = datestr(now,'yyyy');
      | else
      |     last = last(end-3:end);
      | end
      | 
      | if strcmp(first,last)
      |     fprintf('%s -- Copyright %s Nexteer',NxtrConf,first)
      | else
      |     fprintf('%s -- %s%s- %s Nexteer',NxtrConf,char(169),first,last)
      | end
  Max Counts : Constant  Value=2^32-1  OutDataTypeStr=uint32
  Subtract1 : Sum  Inputs=+-+
  Out1 : Outport
  wires:
  Subtract1/1 -> Out1/1
  Max Counts/1 -> Subtract1/1
  ref/1 -> Subtract1/2
  new/1 -> Subtract1/3

== system CF012A_GmStrtStop/GmStrtStop/GmStrtStopPer1/Inter1ToStopModFlg/SpanTi/SetFalse/CopyRight2 ==

== system CF012A_GmStrtStop/GmStrtStop/GmStrtStopPer1/Inter1ToStopModFlg/SpanTi/SetTrue/CopyRight2 ==

== system CF012A_GmStrtStop/GmStrtStop/GmStrtStopPer1/Inter2ToStopModFlg/RefTi/GetRefTmr100MicroSec32bit/CopyRight2 ==

== system CF012A_GmStrtStop/GmStrtStop/GmStrtStopPer1/Inter2ToStopModFlg/SpanTi/GetTiSpan100MicroSec32bit/CopyRight2 ==

== system CF012A_GmStrtStop/GmStrtStop/GmStrtStopPer1/Inter2ToStopModFlg/SpanTi/GetTiSpan100MicroSec32bit/Nowrapping ==
  new : Inport
  ref : Inport  Port=2
  Action Port : ActionPort  ActionType=then
  CopyRight2 : Subsystem  Description=|  mask(Copyright Information){none=on}
      | Copyright info block.                                               
      |                                                                     
      | Place copyright information at the top of every subsystem in design.
      mask prompts: none "No parameters"
      mask help: Place copyright information at the top of every subsystem in design.
      mask Display:
      | NxtrConf = 'Nexteer Confidential';
      | 
      | sys = bdroot; %handle for the current model ("system")
      | first = get_param(sys,'Created');
      | if(isempty(first))
      |     first = datestr(now,'yyyy');
      | else
      |     first = first(end-3:end);  %year is last four digits
      | end
      | 
      | last = get_param(sys,'LastModifiedDate');
      | if isempty(last)
      |     last = datestr(now,'yyyy');
      | else
      |     last = last(end-3:end);
      | end
      | 
      | if strcmp(first,last)
      |     fprintf('%s -- Copyright %s Nexteer',NxtrConf,first)
      | else
      |     fprintf('%s -- %s%s- %s Nexteer',NxtrConf,char(169),first,last)
      | end
  Subtract1 : Sum  Inputs=+-
  Out1 : Outport
  wires:
  ref/1 -> Subtract1/2
  new/1 -> Subtract1/1
  Subtract1/1 -> Out1/1

== system CF012A_GmStrtStop/GmStrtStop/GmStrtStopPer1/Inter2ToStopModFlg/SpanTi/GetTiSpan100MicroSec32bit/Wrapping ==
  new : Inport
  ref : Inport  Port=2
  Action Port : ActionPort  ActionType=else
  CopyRight2 : Subsystem  Description=|  mask(Copyright Information){none=on}
      | Copyright info block.                                               
      |                                                                     
      | Place copyright information at the top of every subsystem in design.
      mask prompts: none "No parameters"
      mask help: Place copyright information at the top of every subsystem in design.
      mask Display:
      | NxtrConf = 'Nexteer Confidential';
      | 
      | sys = bdroot; %handle for the current model ("system")
      | first = get_param(sys,'Created');
      | if(isempty(first))
      |     first = datestr(now,'yyyy');
      | else
      |     first = first(end-3:end);  %year is last four digits
      | end
      | 
      | last = get_param(sys,'LastModifiedDate');
      | if isempty(last)
      |     last = datestr(now,'yyyy');
      | else
      |     last = last(end-3:end);
      | end
      | 
      | if strcmp(first,last)
      |     fprintf('%s -- Copyright %s Nexteer',NxtrConf,first)
      | else
      |     fprintf('%s -- %s%s- %s Nexteer',NxtrConf,char(169),first,last)
      | end
  Max Counts : Constant  Value=2^32-1  OutDataTypeStr=uint32
  Subtract1 : Sum  Inputs=+-+
  Out1 : Outport
  wires:
  new/1 -> Subtract1/3
  ref/1 -> Subtract1/2
  Max Counts/1 -> Subtract1/1
  Subtract1/1 -> Out1/1

== system CF012A_GmStrtStop/GmStrtStop/GmStrtStopPer1/Inter2ToStopModFlg/SpanTi/SetFalse/CopyRight2 ==

== system CF012A_GmStrtStop/GmStrtStop/GmStrtStopPer1/Inter2ToStopModFlg/SpanTi/SetTrue/CopyRight2 ==

== system CF012A_GmStrtStop/GmStrtStop/GmStrtStopPer1/Inter1ToStopModFlg/SpanTi/GetTiSpan100MicroSec32bit/Nowrapping/CopyRight2 ==

== system CF012A_GmStrtStop/GmStrtStop/GmStrtStopPer1/Inter1ToStopModFlg/SpanTi/GetTiSpan100MicroSec32bit/Wrapping/CopyRight2 ==

== system CF012A_GmStrtStop/GmStrtStop/GmStrtStopPer1/Inter2ToStopModFlg/SpanTi/GetTiSpan100MicroSec32bit/Nowrapping/CopyRight2 ==

== system CF012A_GmStrtStop/GmStrtStop/GmStrtStopPer1/Inter2ToStopModFlg/SpanTi/GetTiSpan100MicroSec32bit/Wrapping/CopyRight2 ==

== stateflow chart CF012A_GmStrtStop/GmStrtStop/GmStrtStopPer1/StartStopStateDetermination ==
  state Ena
    state FltModInactv
      state NormMod
        en:
        StrtStopSt=NORMMOD_CNT_U08;
        StrtStopSca=FULLASSISCA_ULS_F32;
      state Inter2Mod
        en:
        StrtStopSt=MOD2_CNT_U08;
        StrtStopSca=GmStrtStopMod2Sca;
      state Inter1Mod
        en:
        StrtStopSt=MOD1_CNT_U08;
        StrtStopSca=GmStrtStopMod1Sca;
      state StopMod
        en:
        StrtStopSt=STOPMOD_CNT_U08;
        StrtStopSca=GmStrtStopStopModSca;
      (default) -> NormMod
      Inter2Mod -> NormMod [order 1] : [VehSpd>=GmStrtStopNormModVehSpdTranThd||...
          | EngSpd>GmStrtStopNormModEngTranThd]
      StopMod -> NormMod [order 1] : [EngSpd > GmStrtStopNormModEngTranThd]
      Inter1Mod -> NormMod [order 1] : [EngSpd>GmStrtStopNormModEngTranThd]
      NormMod -> Inter1Mod : [EngSpd<=GmStrtStopMod1EngTranThd&&...
          | VehSpd<=GmStrtStopMod1VehSpdTranThd]
      Inter2Mod -> StopMod [order 2] : [VehSpd<=GmStrtStopStopMod2VehSpdTranThd && ...
          | abs(HwVel)<=GmStrtStopStopMod2HwVelTranThd && ...
          | abs(HwTq)<=GmStrtStopStopMod2HwTqTranThd&&...
          | TranInter2ToStopMod]
      StopMod -> Inter2Mod [order 2] : [VehSpd>GmStrtStopStopMod2VehSpdTranThd]
      Inter1Mod -> StopMod [order 2] : [VehSpd<=GmStrtStopStopMod1VehSpdTranThd &&...
          | abs(HwVel)<=GmStrtStopStopMod1HwVelTranThd &&...
          | abs(HwTq)<=GmStrtStopStopMod1HwTqTranThd&&...
          | TranInter1ToStopMod]
    state FltModActv
      en:
      StrtStopSt=FLTMOD_CNT_U08;
      StrtStopSca=FULLASSISCA_ULS_F32;
    (default) -> FltModInactv
    FltModInactv -> FltModActv : [FltModEna~=0]
    FltModActv -> NormMod : [FltModEna==0]
  state Di
    StrtStopSt=DISMOD_CNT_U08;
    StrtStopSca=FULLASSISCA_ULS_F32;
  (default) -> (junction 235)
  (junction 235) -> Ena [order 2]
  (junction 235) -> Di [order 1] : [StrtStopEna==0]
  Ena -> Di : [StrtStopEna==0]
  Di -> FltModActv : [StrtStopEna==1 &&...
      | FltModEna==1]
  data: StrtStopEna input; HwTq input; HwVel input; FltModEna input; VehSpd input; EngSpd input; StrtStopSt output uint8; GmStrtStopMod1EngTranThd parameter; GmStrtStopMod1VehSpdTranThd parameter; GmStrtStopMod1Sca parameter; GmStrtStopStopMod1VehSpdTranThd parameter; GmStrtStopStopMod1HwTqTranThd parameter; GmStrtStopStopMod1HwVelTranThd parameter; GmStrtStopStopModSca parameter; GmStrtStopStopMod2VehSpdTranThd parameter; GmStrtStopMod2Sca parameter; GmStrtStopStopMod2HwTqTranThd parameter; GmStrtStopStopMod2HwVelTranThd parameter; GmStrtStopNormModVehSpdTranThd parameter; GmStrtStopNormModEngTranThd parameter; StrtStopSca output single; TranInter2ToStopMod input; TranInter1ToStopMod input; DISMOD_CNT_U08 parameter; FLTMOD_CNT_U08 parameter; MOD1_CNT_U08 parameter; MOD2_CNT_U08 parameter; NORMMOD_CNT_U08 parameter; STOPMOD_CNT_U08 parameter; FULLASSISCA_ULS_F32 parameter
